simulink model "QArm_Workspace_MB_1"  (R2022a)
settings: Solver=ode4  StartTime=0.0  StopTime=inf  FixedStep=1/1000  RelTol=1e-3  EnableMultiTasking=on
model workspace (MAT data in the model file):
  cameraStepSize : Simulink.Parameter (value not decoded)
  mainStepSize : Simulink.Parameter (value not decoded)
symbols that are objects in the model workspace (value not decoded): cameraStepSize, mainStepSize
undefined symbols (not defined in the file): interleaved, RGB
libraries: quarc_library x12, simulink x3
(part 3 of 3)

== matlab function QArm_Workspace_MB_1/Virtual QArm/Manipulator Joint Plant - Queens/Subsystem/forward kinematics ==
  data: phi input size=[4]; p4 output size=[3]; R04 output size=[3,3]
function [p4, R04] = qarmForwardKinematics(phi)

%% QUANSER_ARM_FPK
% v 4.0 - 4th June 2020

% REFERENCE: 
% Chapter 3. Forward Kinematics
% Robot Dynamics and Control 
% Spong, Vidyasagar
% 1989

% INPUTS:
% phi     : Alternate joint angles vector 4 x 1

% OUTPUTS:
% p4      : End-effector frame {4} position vector expressed in base frame {0}
% R04     : rotation matrix from end-effector frame {4} to base frame {0}

%% Manipulator parameters:
L1 = 0.1400;
L2 = 0.3500;
L3 = 0.0500;
L4 = 0.2500;
L5 = 0.1500;

%% Alternate parameters
l1 = L1;
l2 = sqrt(L2^2 + L3^2);
l3 = L4 + L5;
beta = atan(L3/L2);

%% From phi space to theta space 
theta = phi;
theta(1) = phi(1);
theta(2) = phi(2) + beta - pi/2;
theta(3) = phi(3) - beta;
theta(4) = phi(4);

%% Transformation matrices for all frames:

% T{i-1}{i} = quanser_arm_DH(  a, alpha,  d,     theta );
        T01 = quanser_arm_DH(  0, -pi/2, l1,  theta(1) );
        T12 = quanser_arm_DH( l2,     0,  0,  theta(2) );
        T23 = quanser_arm_DH(  0, -pi/2,  0,  theta(3) );
        T34 = quanser_arm_DH(  0,     0, l3,  theta(4) );

        T02 = T01*T12;
        T03 = T02*T23;
        T04 = T03*T34;

%% Position of end-effector Transformation

% Extract the Position vector 
% p1   = T01(1:3,4);
% p2   = T02(1:3,4);
% p3   = T03(1:3,4);
p4   = T04(1:3,4);

% Extract the Rotation matrix
% R01 = T01(1:3,1:3);
% R02 = T02(1:3,1:3);
% R03 = T03(1:3,1:3);
R04 = T04(1:3,1:3);

end

function T = quanser_arm_DH(a,alpha,d,theta)

%% QUANSER_ARM_DH
% v 1.0 - 26th March 2019

% REFERENCE: 
% Chapter 3. Forward and Inverse Kinematics
% Robot Modeling and Control 
% Spong, Hutchinson, Vidyasagar
% 2006

% INPUTS:
% a       :   translation  : along : x_{i}   : from : z_{i-1} : to : z_{i}
% alpha   :      rotation  : about : x_{i}   : from : z_{i-1} : to : z_{i}
% d       :   translation  : along : z_{i-1} : from : x_{i-1} : to : x_{i}
% theta   :      rotation  : about : z_{i-1} : from : x_{i-1} : to : x_{i}
% NOTE: Standard DH Parameters

% OUTPUTS:
% T       : transformation                   : from :     {i} : to : {i-1}

%%
% Rotation Transformation about z axis by theta
T_R_z = [cos(theta) -sin(theta) 0 0;
         sin(theta)  cos(theta) 0 0;
                  0           0 1 0;
                  0           0 0 1];
     
% Translation Transformation along z axis by d
T_T_z = [1 0 0 0;
         0 1 0 0;
         0 0 1 d;
         0 0 0 1];

% Translation Transformation along x axis by a
T_T_x = [1 0 0 a;
         0 1 0 0;
         0 0 1 0;
         0 0 0 1];

% Rotation Transformation about x axis by alpha
T_R_x = [1          0           0 0;
         0 cos(alpha) -sin(alpha) 0;
         0 sin(alpha)  cos(alpha) 0;
         0          0           0 1];

% For a transformation FROM frame {i} TO frame {i-1}: A
T = T_R_z*T_T_z*T_T_x*T_R_x;

end

== matlab function QArm_Workspace_MB_1/To//From Simulation/MATLAB Function1 ==
  data: Receive input size=65537; RequestServerUpdate output; New input; Base output; Shoulder output; Elbow output; Wrist output; Gripper output; StaticEnvCollision output; FingerpadDetection output; EnvironmentReset output; Mass output; TargetLocation output; ActualLocation output
function [RequestServerUpdate, Base, Shoulder, Elbow, Wrist, Gripper, StaticEnvCollision, FingerpadDetection, EnvironmentReset, Mass, TargetLocation, ActualLocation]  = QArmApplicationWorkspaceDecodePacket(Receive, New)

%% Setup

persistent iBase;
persistent iShoulder;
persistent iElbow;
persistent iWrist;
persistent iGripper;
persistent iStaticEnvCollision;
persistent iFingerpadDetection;
persistent iMass;
persistent iTargetLocation;
persistent iActualLocation;

if isempty(iBase)
    iBase = single(0);
    iShoulder = single(0);
    iElbow = single(0);
    iWrist = single(0);
    iGripper = single(0);
    iStaticEnvCollision = uint8(0);
    iFingerpadDetection = [uint8(0); uint8(0); uint8(0); uint8(0)];
    iMass = single(0);
    iTargetLocation = [single(0); single(0); single(0)];
    iActualLocation = [single(0); single(0); single(0)];
end

% Need to assign outputs here even though they are reassigned at the end
% since matlab can't determine the signal widths
Base = single(0);
Shoulder = single(0);
Elbow = single(0);
Wrist = single(0);
Gripper = single(0);
StaticEnvCollision = uint8(0);
FingerpadDetection = [uint8(0); uint8(0); uint8(0); uint8(0)];
EnvironmentReset = 0;
Mass = single(0);
TargetLocation = [single(0); single(0); single(0)];
ActualLocation = [single(0); single(0); single(0)];
NumSegmentsHit = uint8(0);

RequestServerUpdate = 0;
PacketSize = length(Receive);

% Packet > 0, new data, and magic number in first index
if ((PacketSize > 0) && (New == 1) && (Receive(1) == uint8(123)))
    
    %skip magic number
    Index = int32(2);
    
    while(Index <= PacketSize)
       
        %% Get container details
        ContainerSize = typecast(uint8(flip(Receive(Index:Index+3))), 'int32');
        DeviceID = typecast(uint8(flip(Receive(Index+4:Index+7))), 'int32');
        DeviceNum = typecast(uint8(flip(Receive(Index+8:Index+11))), 'int32');
        DeviceFunction = uint8(Receive(Index+12));
        PayloadStart = Index+13;
        PayloadEnd = Index+ContainerSize-1;
        
        %% Pass container to appropriate decoding function
        if (DeviceID == 10) %is this a QArm container?
            
            if (DeviceFunction == 11) %UE4 State Response
                [iBase, iShoulder, iElbow, iWrist, iGripper, iStaticEnvCollision, iFingerpadDetection] = QArmDecodeUE4StateContainer(Receive, PayloadStart);  
                RequestServerUpdate = 1;
            elseif (DeviceFunction == 13) %Mode change
                [iMode] = QArmDecodeModeContainer(Receive, PayloadStart);  
                RequestServerUpdate = 1;
            elseif (DeviceFunction == 51) %Gripper properties
                [ObjectID, iMass, PropertyString] = QArmDecodeGripperObject(Receive, PayloadStart);
                %RequestServerUpdate = 1;
            elseif (DeviceFunction == 61) %Collision spheres
                [iTargetLocation, iActualLocation] = QArmDecodeEndEffectorCollisionSpheres(Receive, PayloadStart);
                %RequestServerUpdate = 1;   
            elseif (DeviceFunction == 71) %Collision segments
                [Yaw, Shoulder, Elbow, Wrist, FingerLP, FingerLD, FingerRP, FingerRD] = QArmDecodeSegmentCollisions(Receive, PayloadStart);
                %RequestServerUpdate = 1; 
                
                NumSegmentsHit = typecast(single(Yaw + Shoulder + Elbow + Wrist + FingerLP + FingerLD + FingerRP + FingerRD), 'uint8');
            end
        
        elseif (DeviceID == 1001) %Simulink notification
            if (DeviceFunction == 200) %Reset button
                EnvironmentReset = 1;
            end
        end
        
        
        
        %% Process next container if any data is left.
        Index = Index+ContainerSize;
    end


end

Base = iBase;
Shoulder = iShoulder;
Elbow = iElbow;
Wrist = iWrist;
Gripper = iGripper;
StaticEnvCollision = iStaticEnvCollision;
FingerpadDetection = iFingerpadDetection;
Mass = iMass;
ActualLocation = iActualLocation;
TargetLocation = iTargetLocation;

== matlab function QArm_Workspace_MB_1/To//From Simulation/MATLAB Function ==
  settings: updateMethod=DISCRETE  sampleTime=qc_get_step_size
  data: Packet output size=65537; ServerState input; SendStateUpdate input; Enable output; DeviceNumber input; Base input; Shoulder input; Elbow input; Wrist input; Gripper input; BaseColor_v3 input; ArmBrightness input
function [Packet,Enable] = QArmApplicationWorkspaceMakePacket(ServerState, SendStateUpdate, DeviceNumber, Base, Shoulder, Elbow, Wrist, Gripper, BaseColor_v3, ArmBrightness) 

% Be sure to set the maximum signal size of the variable size Packet port 
% in Simulink->Edit Data of the editor window.  Size should be 65537 or
% larger to ensure that the stream server generates a 4 byte packet size.

%% Setup
persistent LastServerState;

if isempty(LastServerState)
    LastServerState = uint8(0);
end

Enable = 0;
Packet = uint8([]);

%% On connection
if ((ServerState == 2) && (LastServerState ~= 2))
    Packet = QArmMakeCommandStateContainer(DeviceNumber, Base, Shoulder, Elbow, Wrist, Gripper, BaseColor_v3, ArmBrightness); 
    Packet = [Packet; QArmMakeRequestGripperObject(DeviceNumber)];
    Packet = [Packet; QArmMakeRequestEndEffectorCollisionSpheres(DeviceNumber)];
    Packet = [Packet; QArmMakeRequestSegmentCollisions(DeviceNumber)];
end

%% Send new State Container
% Previous state processed, send a new one
if (SendStateUpdate)
    Packet = QArmMakeCommandStateContainer(DeviceNumber, Base, Shoulder, Elbow, Wrist, Gripper, BaseColor_v3, ArmBrightness); 
    Packet = [Packet; QArmMakeRequestGripperObject(DeviceNumber)];
    Packet = [Packet; QArmMakeRequestEndEffectorCollisionSpheres(DeviceNumber)];
    Packet = [Packet; QArmMakeRequestSegmentCollisions(DeviceNumber)];
end

%% Transmit
% If we have data to send, enable the transmit
PacketLength = length(Packet);

if (PacketLength > 0)
    % Add magic byte.  This is just for error handling and isn't typically
    % required in simulink, but useful in lower-level languages like Python
    Packet = [uint8(123); Packet];
    
    Enable = 1; 
end


LastServerState = ServerState;

== matlab function QArm_Workspace_MB_1/Virtual QArm/Manipulator Joint Plants/Subsystem/forward kinematics ==
  data: phi input size=[4]; p4 output size=[3]; R04 output size=[3,3]
function [p4, R04] = qarmForwardKinematics(phi)

%% QUANSER_ARM_FPK
% v 4.0 - 4th June 2020

% REFERENCE: 
% Chapter 3. Forward Kinematics
% Robot Dynamics and Control 
% Spong, Vidyasagar
% 1989

% INPUTS:
% phi     : Alternate joint angles vector 4 x 1

% OUTPUTS:
% p4      : End-effector frame {4} position vector expressed in base frame {0}
% R04     : rotation matrix from end-effector frame {4} to base frame {0}

%% Manipulator parameters:
L1 = 0.1400;
L2 = 0.3500;
L3 = 0.0500;
L4 = 0.2500;
L5 = 0.1500;

%% Alternate parameters
l1 = L1;
l2 = sqrt(L2^2 + L3^2);
l3 = L4 + L5;
beta = atan(L3/L2);

%% From phi space to theta space 
theta = phi;
theta(1) = phi(1);
theta(2) = phi(2) + beta - pi/2;
theta(3) = phi(3) - beta;
theta(4) = phi(4);

%% Transformation matrices for all frames:

% T{i-1}{i} = quanser_arm_DH(  a, alpha,  d,     theta );
        T01 = quanser_arm_DH(  0, -pi/2, l1,  theta(1) );
        T12 = quanser_arm_DH( l2,     0,  0,  theta(2) );
        T23 = quanser_arm_DH(  0, -pi/2,  0,  theta(3) );
        T34 = quanser_arm_DH(  0,     0, l3,  theta(4) );

        T02 = T01*T12;
        T03 = T02*T23;
        T04 = T03*T34;

%% Position of end-effector Transformation

% Extract the Position vector 
% p1   = T01(1:3,4);
% p2   = T02(1:3,4);
% p3   = T03(1:3,4);
p4   = T04(1:3,4);

% Extract the Rotation matrix
% R01 = T01(1:3,1:3);
% R02 = T02(1:3,1:3);
% R03 = T03(1:3,1:3);
R04 = T04(1:3,1:3);

end

function T = quanser_arm_DH(a,alpha,d,theta)

%% QUANSER_ARM_DH
% v 1.0 - 26th March 2019

% REFERENCE: 
% Chapter 3. Forward and Inverse Kinematics
% Robot Modeling and Control 
% Spong, Hutchinson, Vidyasagar
% 2006

% INPUTS:
% a       :   translation  : along : x_{i}   : from : z_{i-1} : to : z_{i}
% alpha   :      rotation  : about : x_{i}   : from : z_{i-1} : to : z_{i}
% d       :   translation  : along : z_{i-1} : from : x_{i-1} : to : x_{i}
% theta   :      rotation  : about : z_{i-1} : from : x_{i-1} : to : x_{i}
% NOTE: Standard DH Parameters

% OUTPUTS:
% T       : transformation                   : from :     {i} : to : {i-1}

%%
% Rotation Transformation about z axis by theta
T_R_z = [cos(theta) -sin(theta) 0 0;
         sin(theta)  cos(theta) 0 0;
                  0           0 1 0;
                  0           0 0 1];
     
% Translation Transformation along z axis by d
T_T_z = [1 0 0 0;
         0 1 0 0;
         0 0 1 d;
         0 0 0 1];

% Translation Transformation along x axis by a
T_T_x = [1 0 0 a;
         0 1 0 0;
         0 0 1 0;
         0 0 0 1];

% Rotation Transformation about x axis by alpha
T_R_x = [1          0           0 0;
         0 cos(alpha) -sin(alpha) 0;
         0 sin(alpha)  cos(alpha) 0;
         0          0           0 1];

% For a transformation FROM frame {i} TO frame {i-1}: A
T = T_R_z*T_T_z*T_T_x*T_R_x;

end

== matlab function QArm_Workspace_MB_1/To//From Simulation/MATLAB Function2 ==
  settings: updateMethod=DISCRETE  sampleTime=mainStepSize
  data: Packet output size=65537; ServerState input; SendStateUpdate input; Enable output; DeviceNumber input; Clock input; Threshold input; Disable_RGB input; Disable_Depth input
function [Packet,Enable] = QArmApplicationWorkspaceMakeVideoPacketData(ServerState, SendStateUpdate, DeviceNumber, Clock, Threshold, Disable_RGB, Disable_Depth) 

% Be sure to set the maximum signal size of the variable size Packet port 
% in Simulink->Edit Data of the editor window.  Size should be 65537 or
% larger to ensure that the stream server generates a 4 byte packet size.

%% Setup
persistent LastServerState;
persistent timeLastSend;
persistent readyToSend;

if isempty(LastServerState)
    LastServerState = uint8(0);
    readyToSend = uint8(0);
    timeLastSend = -Threshold;
end

Enable = 0;
Packet = uint8([]);

%% On connection
if ((ServerState == 2) && (LastServerState ~= 2))
    if (Disable_RGB == 0)
        Packet = QArmMakeRGBRequestContainer(DeviceNumber);
    end
    
    if (Disable_Depth == 0)
        Packet = [Packet; QArmMakeDepthRequestContainer(DeviceNumber)];
    end
    
    if ((Disable_RGB == 1) && (Disable_Depth == 1))
        % Do this to keep the server connection alive and avoid the
        % reconnection overhead
        Packet = QArmMakePingRequestContainer(DeviceNumber);
    end

end

%% Send new State Container
% Previous state processed, send a new one
if (SendStateUpdate)
    readyToSend = uint8(1);
end

if readyToSend && ((Clock - timeLastSend) > Threshold)
    if (Disable_RGB == 0)
        Packet = QArmMakeRGBRequestContainer(DeviceNumber);
    end
    
    if (Disable_Depth == 0)
        Packet = [Packet; QArmMakeDepthRequestContainer(DeviceNumber)];
    end
    
    if ((Disable_RGB == 1) && (Disable_Depth == 1))
        % Do this to keep the server connection alive and avoid the
        % reconnection overhead
        Packet = QArmMakePingRequestContainer(DeviceNumber);
    end    
    readyToSend = uint8(0);
    timeLastSend = Clock;
end


%% Transmit
% If we have data to send, enable the transmit
PacketLength = length(Packet);

if (PacketLength > 0)
    % Add magic byte.  This is just for error handling and isn't typically
    % required in simulink, but useful in lower-level languages like Python
    Packet = [uint8(123); Packet];
    
    Enable = 1; 
end

LastServerState = ServerState;

== matlab function QArm_Workspace_MB_1/To//From Simulation/Collision/forward kinematics ==
  data: phi input; p4 output; R04 output
function [p4, R04] = qarmForwardKinematics(phi)

%% QUANSER_ARM_FPK
% v 4.0 - 4th June 2020

% REFERENCE: 
% Chapter 3. Forward Kinematics
% Robot Dynamics and Control 
% Spong, Vidyasagar
% 1989

% INPUTS:
% phi     : Alternate joint angles vector 4 x 1

% OUTPUTS:
% p4      : End-effector frame {4} position vector expressed in base frame {0}
% R04     : rotation matrix from end-effector frame {4} to base frame {0}

%% Manipulator parameters:
L1 = 0.1400;
L2 = 0.3500;
L3 = 0.0500;
L4 = 0.2500;
L5 = 0.1500;

%% Alternate parameters
l1 = L1;
l2 = sqrt(L2^2 + L3^2);
l3 = L4 + L5;
beta = atan(L3/L2);

%% From phi space to theta space 
theta = phi;
theta(1) = phi(1);
theta(2) = phi(2) + beta - pi/2;
theta(3) = phi(3) - beta;
theta(4) = phi(4);

%% Transformation matrices for all frames:

% T{i-1}{i} = quanser_arm_DH(  a, alpha,  d,     theta );
        T01 = quanser_arm_DH(  0, -pi/2, l1,  theta(1) );
        T12 = quanser_arm_DH( l2,     0,  0,  theta(2) );
        T23 = quanser_arm_DH(  0, -pi/2,  0,  theta(3) );
        T34 = quanser_arm_DH(  0,     0, l3,  theta(4) );

        T02 = T01*T12;
        T03 = T02*T23;
        T04 = T03*T34;

%% Position of end-effector Transformation

% Extract the Position vector 
% p1   = T01(1:3,4);
% p2   = T02(1:3,4);
% p3   = T03(1:3,4);
p4   = T04(1:3,4);

% Extract the Rotation matrix
% R01 = T01(1:3,1:3);
% R02 = T02(1:3,1:3);
% R03 = T03(1:3,1:3);
R04 = T04(1:3,1:3);

end

function T = quanser_arm_DH(a,alpha,d,theta)

%% QUANSER_ARM_DH
% v 1.0 - 26th March 2019

% REFERENCE: 
% Chapter 3. Forward and Inverse Kinematics
% Robot Modeling and Control 
% Spong, Hutchinson, Vidyasagar
% 2006

% INPUTS:
% a       :   translation  : along : x_{i}   : from : z_{i-1} : to : z_{i}
% alpha   :      rotation  : about : x_{i}   : from : z_{i-1} : to : z_{i}
% d       :   translation  : along : z_{i-1} : from : x_{i-1} : to : x_{i}
% theta   :      rotation  : about : z_{i-1} : from : x_{i-1} : to : x_{i}
% NOTE: Standard DH Parameters

% OUTPUTS:
% T       : transformation                   : from :     {i} : to : {i-1}

%%
% Rotation Transformation about z axis by theta
T_R_z = [cos(theta) -sin(theta) 0 0;
         sin(theta)  cos(theta) 0 0;
                  0           0 1 0;
                  0           0 0 1];
     
% Translation Transformation along z axis by d
T_T_z = [1 0 0 0;
         0 1 0 0;
         0 0 1 d;
         0 0 0 1];

% Translation Transformation along x axis by a
T_T_x = [1 0 0 a;
         0 1 0 0;
         0 0 1 0;
         0 0 0 1];

% Rotation Transformation about x axis by alpha
T_R_x = [1          0           0 0;
         0 cos(alpha) -sin(alpha) 0;
         0 sin(alpha)  cos(alpha) 0;
         0          0           0 1];

% For a transformation FROM frame {i} TO frame {i-1}: A
T = T_R_z*T_T_z*T_T_x*T_R_x;

end

== matlab function QArm_Workspace_MB_1/Virtual QArm/Manipulator Joint Plants/Subsystem/forward differential kinematics ==
  data: phi input size=[4]; J output size=[4,4]
function J  = qarmDifferentialKinematics(phi)

%% QUANSER_ARM_FPK
% v 4.0 - 4th June 2020

% REFERENCE: 
% Chapter 3. Forward Kinematics
% Robot Dynamics and Control 
% Spong, Vidyasagar
% 1989

% INPUTS:
% phi     : Alternate joint angles vector 4 x 1

% OUTPUTS:
% p4      : End-effector frame {4} position vector expressed in base frame {0}
% R04     : rotation matrix from end-effector frame {4} to base frame {0}

%% Manipulator parameters:
L1 = 0.1400;
L2 = 0.3500;
L3 = 0.0500;
L4 = 0.2500;
L5 = 0.1500;

%% Alternate parameters
l1 = L1;
l2 = sqrt(L2^2 + L3^2);
l3 = L4 + L5;
beta = atan(L3/L2);

%% From phi space to theta space 
theta = phi;
theta(1) = phi(1);
theta(2) = phi(2) + beta - pi/2;
theta(3) = phi(3) - beta;
theta(4) = phi(4);

%% Transformation matrices for all frames:

J = eye(4);
J(1,1) = - l2*sin(theta(1))*cos(theta(2)) + l3*sin(theta(1))*sin(theta(2)+theta(3)); 
J(1,2) = - l2*cos(theta(1))*sin(theta(2)) - l3*cos(theta(1))*cos(theta(2)+theta(3)); 
J(1,3) = - l3*cos(theta(1))*cos(theta(2)+theta(3)); 
J(1,4) = 0;
J(2,1) =   l2*cos(theta(1))*cos(theta(2)) - l3*cos(theta(1))*sin(theta(2)+theta(3)); 
J(2,2) = - l2*sin(theta(1))*sin(theta(2)) - l3*sin(theta(1))*cos(theta(2)+theta(3)); 
J(2,3) = - l3*sin(theta(1))*cos(theta(2)+theta(3));
J(2,4) = 0;
J(3,1) = 0; 
J(3,2) = - l2*cos(theta(2)) + l3*sin(theta(2)+theta(3)); 
J(3,3) =   l3*sin(theta(2)+theta(3));
J(3,4) = 0;
J(4,1) = 0;
J(4,2) = 0;
J(4,3) = 0;
J(4,4) = 1;

end
